simulink model "CSTR_MalhaAberta"  (R2021a)
settings: Solver=VariableStepAuto  StartTime=0.0  StopTime=10.0  RelTol=1e-3
values from neighbouring files (symbols this model uses):
  caf = 10    [mainCSTR.m]    (also in mainCSTR_control.m; mainControlCSTR.m; simulation_04_04_2024.mat)
  deltaE = 11843    [mainCSTR.m]    (also in mainCSTR_control.m; mainControlCSTR.m; simulation_04_04_2024.mat)
  deltaH = 5960    [mainCSTR.m]    (also in mainCSTR_control.m; mainControlCSTR.m; simulation_04_04_2024.mat)
  k0 = 9703*3600    (= 34930800)    [mainCSTR.m]    (also in mainCSTR_control.m; mainControlCSTR.m; simulation_04_04_2024.mat)
  R = 1.987    [mainCSTR.m]    (also in mainCSTR_control.m; mainControlCSTR.m; rga.m = pinv(G.').*G; simulation_04_04_2024.mat)
  rhocp = 500    [mainCSTR.m]    (also in mainCSTR_control.m; mainControlCSTR.m; simulation_04_04_2024.mat)
  Tf = 298    [mainCSTR.m]    (also in mainCSTR_control.m; mainControlCSTR.m; simulation_04_04_2024.mat)
  UAoV = 150    [mainCSTR.m]    (also in mainCSTR_control.m; mainControlCSTR.m; simulation_04_04_2024.mat)
  x0model = [5, 350]    [mainCSTR.m]    (also in mainCSTR_control.m = [8.5636  311.1710]; mainControlCSTR.m = [8.5636  311.1706]; simulation_04_04_2024.mat = [5 350])
settings Model: Creator=Aula  LastModifiedBy=Aula

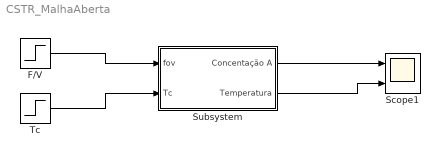
== system CSTR_MalhaAberta ==
  F/V : Step  Time=0  SampleTime=0
  Scope1 : Scope  NumInputPorts=2
  Subsystem : Subsystem
  Tc : Step  Time=0  After=298  SampleTime=0
  wires:
  Subsystem/1(Concentação A) -> Scope1/1
  Subsystem/2(Temperatura) -> Scope1/2
  F/V/1 -> Subsystem/1(fov)
  Tc/1 -> Subsystem/2(Tc)

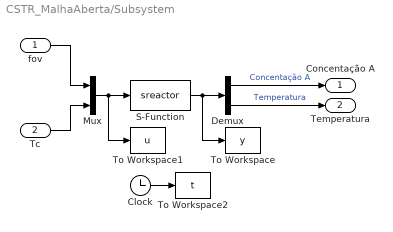
== system CSTR_MalhaAberta/Subsystem ==
  fov : Inport
  Tc : Inport  Port=2
  Clock : Clock
  Demux : Demux  Outputs=2
  Mux : Mux  Inputs=2
  S-Function : S-Function  FunctionName=sreactor  Parameters=x0model,k0,deltaE,R,caf,Tf,deltaH,rhocp,UAoV  SFunctionDeploymentMode=off  EnableBusSupport=off
  To Workspace : ToWorkspace  VariableName=y  SampleTime=0.1
  "To Workspace1 " : ToWorkspace  VariableName=u  SampleTime=-1
  "To Workspace2 " : ToWorkspace  VariableName=t  SampleTime=-1
  Concentação A : Outport
  Temperatura : Outport  Port=2
  wires:
  S-Function/1 -> To Workspace/1, Demux/1
  Clock/1 -> "To Workspace2 "/1
  fov/1 -> Mux/1
  Mux/1 -> "To Workspace1 "/1, S-Function/1
  Tc/1 -> Mux/2
  Demux/2 -> Temperatura/1  "Temperatura"
  Demux/1 -> Concentação A/1  "Concentação A"
